simulink library "generator_lib"  (Simulink 7.8)
settings: Solver=ode45  StartTime=0.0  StopTime=10.0  RelTol=1e-3
undefined symbols (not defined in the file): dfilt, DiscIntNeverNeededParam, fdesignblkfcn, gcbh, ph, Ts
libraries: simulink x91, rtio_opalrt_common x84, powerlib x51, simulink_extras x21, discretizing x14, rteventslib x14, dsparch4 x14, powerlib_extras x4
(part 2 of 10)

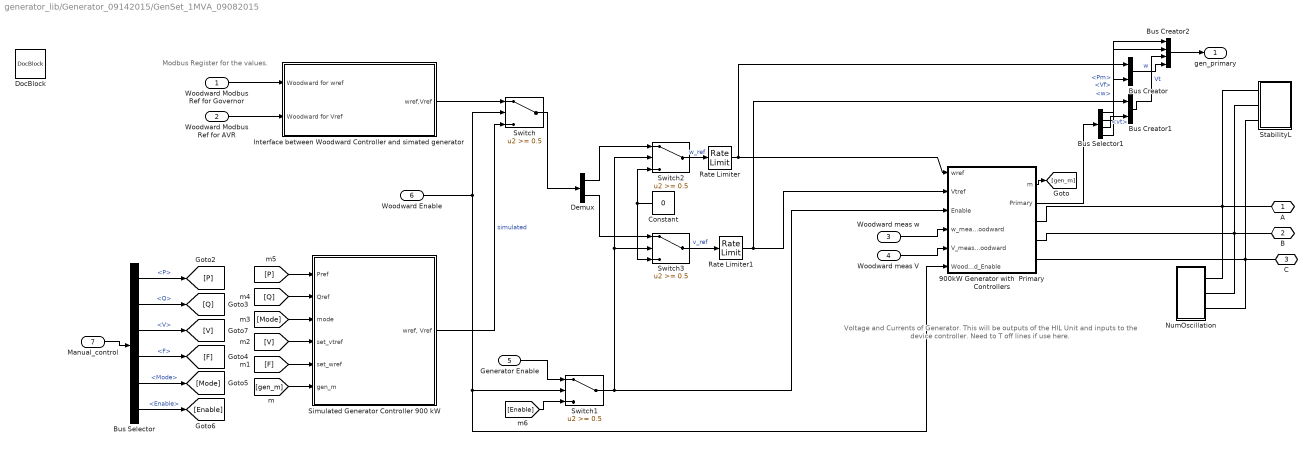
== system generator_lib/Generator_09142015/GenSet_1MVA_09082015 ==
  note: Voltage and Currents of Generator.
      | This will be outputs of the HIL Unit
      | and inputs to the device controller.
      | Need to T off lines if use here.
  note: Modbus Register for the values.
  Woodward Modbus Ref for Governor : Inport
  Woodward Modbus Ref for AVR : Inport  Port=2
  Woodward meas w : Inport  Port=3
  Woodward meas V : Inport  Port=4
  Generator Enable : Inport  Port=5
  Woodward Enable : Inport  Port=6
  Manual_control : Inport  Port=7
  900kW Generator with  Primary Controllers : Subsystem
  Bus Creator : BusCreator  Inputs=2
  Bus Creator1 : BusCreator  Inputs=2
  Bus Creator2 : BusCreator
  Bus Selector : BusSelector  OutputSignals=P,Q,V,F,Mode,Enable
  Bus Selector1 : BusSelector  OutputSignals=Pm,Vf,vt,w
  Constant : Constant  Value=0
  Demux : Demux  Outputs=2
  DocBlock : simulink/Model-Wide Utilities/DocBlock  DocumentType=Text
  Interface between Woodward Controller and simated generator : Subsystem
  NumOscillation : Subsystem
  Rate Limiter : RateLimiter  RisingSlewLimit=0.5  FallingSlewLimit=-0.5  SampleTimeMode=inherited
  Rate Limiter1 : RateLimiter  RisingSlewLimit=0.5  FallingSlewLimit=-0.5  SampleTimeMode=inherited
  Simulated Generator Controller 900 kW : Subsystem
  StabilityL : Subsystem  mask{v=460, kVA=50, pf=1}
  Switch{,1..3} (4 alike) : Switch  Threshold=0.5
  A : PMIOPort  Port=1  Side=Right
  B : PMIOPort  Port=2  Side=Right
  C : PMIOPort  Port=3  Side=Right
  gen_primary : Outport
  wires:
  Woodward Enable/1 -> 900kW Generator with  Primary Controllers/6(Woodward_Enable), Switch1/2, Switch/2
  Rate Limiter1/1 -> Bus Creator1/1, 900kW Generator with  Primary Controllers/2(Vtref)
  Rate Limiter/1 -> Bus Creator/1, 900kW Generator with  Primary Controllers/1(wref)
  Bus Creator2/1 -> gen_primary/1
  Bus Creator/1 -> Bus Creator2/4  "w"
  Bus Creator1/1 -> Bus Creator2/3  "Vt"
  Bus Selector1/1 -> Bus Creator2/1  "<Pm>"
  Bus Selector1/2 -> Bus Creator2/2  "<Vf>"
  Bus Selector1/4 -> Bus Creator/2  "<w>"
  Bus Selector1/3 -> Bus Creator1/2  "<vt>"
  Switch3/1 -> Rate Limiter1/1  "v_ref"
  Constant/1 -> Switch2/3, Switch3/3
  Demux/2 -> Switch3/1
  Demux/1 -> Switch2/1
  Switch2/1 -> Rate Limiter/1  "w_ref"
  Switch1/1 -> Switch3/2, Switch2/2, 900kW Generator with  Primary Controllers/3(Enable)
  [Enable] -> Switch1/3
  Generator Enable/1 -> Switch1/1
  900kW Generator with  Primary Controllers/2(Primary) -> Bus Selector1/1
  Bus Selector/6 -> [Enable]  "<Enable>"
  Woodward meas V/1 -> 900kW Generator with  Primary Controllers/5(V_meas_Woodward)
  Woodward meas w/1 -> 900kW Generator with  Primary Controllers/4(w_meas_Woodward)
  Woodward Modbus Ref for AVR/1 -> Interface between Woodward Controller and simated generator/2(Woodward for Vref)
  Woodward Modbus Ref for Governor/1 -> Interface between Woodward Controller and simated generator/1(Woodward for wref)
  Switch/1 -> Demux/1
  Interface between Woodward Controller and simated generator/1(wref,Vref) -> Switch/1
  900kW Generator with  Primary Controllers/1(m) -> [gen_m]
  Simulated Generator Controller 900 kW/1("wref, Vref") -> Switch/3  "simulated"
  Manual_control/1 -> Bus Selector/1
  Bus Selector/1 -> [P]  "<P>"
  Bus Selector/2 -> [Q]  "<Q>"
  Bus Selector/3 -> [V]  "<V>"
  Bus Selector/4 -> [F]  "<F>"
  Bus Selector/5 -> [Mode]  "<Mode>"
  [gen_m] -> Simulated Generator Controller 900 kW/6(gen_m)
  [P] -> Simulated Generator Controller 900 kW/1(Pref)
  [Q] -> Simulated Generator Controller 900 kW/2(Qref)
  [Mode] -> Simulated Generator Controller 900 kW/3(mode)
  [V] -> Simulated Generator Controller 900 kW/4(set_vtref)
  [F] -> Simulated Generator Controller 900 kW/5(set_wref)
  connections:
  NumOscillation/LConn3 -- 900kW Generator with  Primary Controllers/RConn3 -- C/RConn1 -- StabilityL/LConn3
  NumOscillation/LConn2 -- B/RConn1 -- 900kW Generator with  Primary Controllers/RConn2 -- StabilityL/LConn2
  NumOscillation/LConn1 -- 900kW Generator with  Primary Controllers/RConn1 -- A/RConn1 -- StabilityL/LConn1

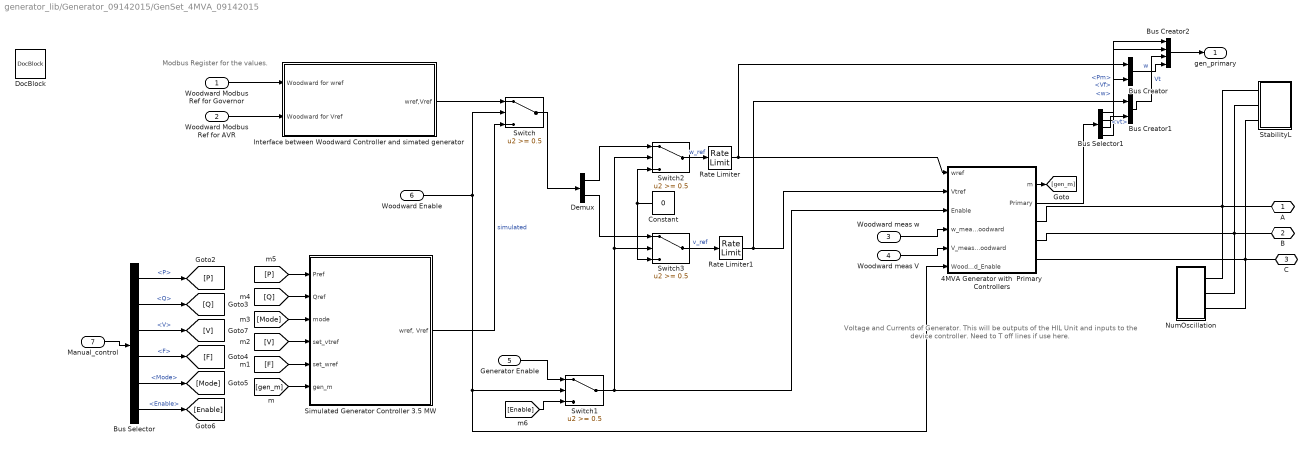
== system generator_lib/Generator_09142015/GenSet_4MVA_09142015 ==
  note: Voltage and Currents of Generator.
      | This will be outputs of the HIL Unit
      | and inputs to the device controller.
      | Need to T off lines if use here.
  note: Modbus Register for the values.
  Woodward Modbus Ref for Governor : Inport
  Woodward Modbus Ref for AVR : Inport  Port=2
  Woodward meas w : Inport  Port=3
  Woodward meas V : Inport  Port=4
  Generator Enable : Inport  Port=5
  Woodward Enable : Inport  Port=6
  Manual_control : Inport  Port=7
  4MVA Generator with  Primary Controllers : Subsystem
  Bus Creator : BusCreator  Inputs=2
  Bus Creator1 : BusCreator  Inputs=2
  Bus Creator2 : BusCreator
  Bus Selector : BusSelector  OutputSignals=P,Q,V,F,Mode,Enable
  Bus Selector1 : BusSelector  OutputSignals=Pm,Vf,vt,w
  Constant : Constant  Value=0
  Demux : Demux  Outputs=2
  DocBlock : simulink/Model-Wide Utilities/DocBlock  DocumentType=Text
  Interface between Woodward Controller and simated generator : Subsystem
  NumOscillation : Subsystem
  Rate Limiter : RateLimiter  RisingSlewLimit=0.5  FallingSlewLimit=-0.5  SampleTimeMode=inherited
  Rate Limiter1 : RateLimiter  RisingSlewLimit=0.5  FallingSlewLimit=-0.5  SampleTimeMode=inherited
  Simulated Generator Controller 3.5 MW : Subsystem
  StabilityL : Subsystem  mask{v=13800, kVA=300, pf=1}
  Switch{,1..3} (4 alike) : Switch  Threshold=0.5
  A : PMIOPort  Port=1  Side=Right
  B : PMIOPort  Port=2  Side=Right
  C : PMIOPort  Port=3  Side=Right
  gen_primary : Outport
  wires:
  Woodward Enable/1 -> 4MVA Generator with  Primary Controllers/6(Woodward_Enable), Switch1/2, Switch/2
  Rate Limiter1/1 -> Bus Creator1/1, 4MVA Generator with  Primary Controllers/2(Vtref)
  Rate Limiter/1 -> Bus Creator/1, 4MVA Generator with  Primary Controllers/1(wref)
  Bus Creator2/1 -> gen_primary/1
  Bus Creator/1 -> Bus Creator2/4  "w"
  Bus Creator1/1 -> Bus Creator2/3  "Vt"
  Bus Selector1/1 -> Bus Creator2/1  "<Pm>"
  Bus Selector1/2 -> Bus Creator2/2  "<Vf>"
  Bus Selector1/4 -> Bus Creator/2  "<w>"
  Bus Selector1/3 -> Bus Creator1/2  "<vt>"
  Switch3/1 -> Rate Limiter1/1  "v_ref"
  Constant/1 -> Switch2/3, Switch3/3
  Demux/2 -> Switch3/1
  Demux/1 -> Switch2/1
  Switch2/1 -> Rate Limiter/1  "w_ref"
  Switch1/1 -> Switch3/2, Switch2/2, 4MVA Generator with  Primary Controllers/3(Enable)
  [Enable] -> Switch1/3
  Generator Enable/1 -> Switch1/1
  4MVA Generator with  Primary Controllers/2(Primary) -> Bus Selector1/1
  Bus Selector/6 -> [Enable]  "<Enable>"
  Woodward meas V/1 -> 4MVA Generator with  Primary Controllers/5(V_meas_Woodward)
  Woodward meas w/1 -> 4MVA Generator with  Primary Controllers/4(w_meas_Woodward)
  Woodward Modbus Ref for AVR/1 -> Interface between Woodward Controller and simated generator/2(Woodward for Vref)
  Woodward Modbus Ref for Governor/1 -> Interface between Woodward Controller and simated generator/1(Woodward for wref)
  Switch/1 -> Demux/1
  Interface between Woodward Controller and simated generator/1(wref,Vref) -> Switch/1
  4MVA Generator with  Primary Controllers/1(m) -> [gen_m]
  Simulated Generator Controller 3.5 MW/1("wref, Vref") -> Switch/3  "simulated"
  Manual_control/1 -> Bus Selector/1
  Bus Selector/1 -> [P]  "<P>"
  Bus Selector/2 -> [Q]  "<Q>"
  Bus Selector/3 -> [V]  "<V>"
  Bus Selector/4 -> [F]  "<F>"
  Bus Selector/5 -> [Mode]  "<Mode>"
  [gen_m] -> Simulated Generator Controller 3.5 MW/6(gen_m)
  [P] -> Simulated Generator Controller 3.5 MW/1(Pref)
  [Q] -> Simulated Generator Controller 3.5 MW/2(Qref)
  [Mode] -> Simulated Generator Controller 3.5 MW/3(mode)
  [V] -> Simulated Generator Controller 3.5 MW/4(set_vtref)
  [F] -> Simulated Generator Controller 3.5 MW/5(set_wref)
  connections:
  NumOscillation/LConn3 -- 4MVA Generator with  Primary Controllers/RConn3 -- C/RConn1 -- StabilityL/LConn3
  NumOscillation/LConn2 -- B/RConn1 -- 4MVA Generator with  Primary Controllers/RConn2 -- StabilityL/LConn2
  NumOscillation/LConn1 -- 4MVA Generator with  Primary Controllers/RConn1 -- A/RConn1 -- StabilityL/LConn1

== system generator_lib/Generator_09142015/Woodward Inputs ==
  note: There will need to be a
      | new scaling factor to use
      | the current cards (0-1A)
  note: GR1 A AOUT (CH00-15)
  note: For 120 => 12Vout / 170Vpk
      | For 480 => 12Vout / 391Vpk
      | For 13.8kv => 12Vout / 11268Vpk
  note: 6Vout / ( 900,000W / 391 Vpk)
  MPU1_speed : Inport
  Generator1_Voltage : Inport  Port=2
  Generator1_Current : Inport  Port=3
  Mains1_Voltage : Inport  Port=4
  Mains1_Current : Inport  Port=5
  MPU2_speed : Inport  Port=6
  Generator2_Voltage : Inport  Port=7
  Generator2_Current : Inport  Port=8
  Mains2_Voltage : Inport  Port=9
  Mains2_Current : Inport  Port=10
  AnalogOut : rtio_opalrt_common/AnalogOut  CtrlName='OpCtrl'  portNb=1  FcnNos=Slot 1 Module A Subsection 1  size=16  maxcount=8  count=8  numchan=8  israngeinput=off  voltagerange=[-16 ... 16]  slot=0  side=0  mismatch=0  slotside=Slot_1_Module_A
      settings: AttributesFormatString=%<CtrlName>
  AnalogOut1 : rtio_opalrt_common/AnalogOut  CtrlName='OpCtrl'  portNb=2  FcnNos=Slot 1 Module A Subsection 2  size=16  maxcount=8  count=8  numchan=8  israngeinput=off  voltagerange=[-16 ... 16]  slot=0  side=0  mismatch=0  slotside=Slot_1_Module_A
      settings: AttributesFormatString=%<CtrlName>
  AnalogOut2 : rtio_opalrt_common/AnalogOut  CtrlName='OpCtrl'  portNb=3  FcnNos=Slot 2 Module A Subsection 1  size=16  maxcount=8  count=8  numchan=8  israngeinput=off  voltagerange=[-16 ... 16]  slot=1  side=0  mismatch=0  slotside=Slot_2_Module_A
      settings: AttributesFormatString=%<CtrlName>
  AnalogOut3 : rtio_opalrt_common/AnalogOut  CtrlName='OpCtrl'  portNb=4  FcnNos=Slot 2 Module A Subsection 2  size=16  maxcount=8  count=8  numchan=8  israngeinput=off  voltagerange=[-16 ... 16]  slot=1  side=0  mismatch=0  slotside=Slot_2_Module_A
      settings: AttributesFormatString=%<CtrlName>
  Demux : Demux  Outputs=2
  Demux{1..5,7..9} (8 alike) : Demux  Outputs=3
  Demux6 : Demux  Outputs=2
  Gain : Gain  Gain=15/391
  Gain1 : Gain  Gain=15/11268
  Gain2 : Gain  Gain=15/(900000/391)
  Gain3 : Gain  Gain=15/(900000/11268)
  Gain4 : Gain  Gain=15/11268
  Gain5 : Gain  Gain=15/11268
  Gain6 : Gain  Gain=15/(900000/391)
  Gain7 : Gain  Gain=15/(900000/11268)
  Mux{,1,3..4} (4 alike) : Mux  Inputs=8
  Mux2 : Mux  Inputs=2
  Mux5 : Mux  Inputs=2
  Speed_System : Subsystem
  Speed_System1 : Subsystem
  Terminator{,1..3} (4 alike) : Terminator
  wires:
  Demux9/3 -> Mux3/8
  Demux9/2 -> Mux3/7
  Demux9/1 -> Mux3/6
  Gain6/1 -> Demux9/1
  Demux8/1 -> Mux3/5
  Gain7/1 -> Demux8/1
  Mains2_Current/1 -> Gain7/1
  Generator2_Current/1 -> Gain6/1
  Speed_System1/1(Out1) -> Mux1/6
  MPU2_speed/1 -> Speed_System1/1(In1)
  Generator2_Voltage/1 -> Gain4/1
  Mains2_Voltage/1 -> Gain5/1
  Gain4/1 -> Demux4/1
  Gain5/1 -> Demux5/1
  Demux7/1 -> Mux3/1
  Gain3/1 -> Demux7/1
  Mains1_Current/1 -> Gain3/1
  Demux3/3 -> Mux3/4
  Demux3/2 -> Mux3/3
  Demux3/1 -> Mux3/2
  Gain2/1 -> Demux3/1
  AnalogOut2/1 -> Terminator2/1
  AnalogOut3/1 -> Terminator3/1
  Demux6/1 -> AnalogOut2/1
  Demux6/2 -> AnalogOut3/1
  Mux3/1 -> Mux5/1
  Mux4/1 -> Mux5/2
  Mux5/1 -> Demux6/1
  Demux5/3 -> Mux1/4
  Demux5/2 -> Mux1/3
  Demux5/1 -> Mux1/2
  Demux4/3 -> Mux1/1
  Demux4/2 -> Mux/8
  Demux4/1 -> Mux/7
  Speed_System/1(Out1) -> Mux1/5
  Demux2/3 -> Mux/6
  Demux2/2 -> Mux/5
  Demux2/1 -> Mux/4
  Demux1/3 -> Mux/3
  Demux1/2 -> Mux/2
  Demux1/1 -> Mux/1
  AnalogOut/1 -> Terminator/1
  AnalogOut1/1 -> Terminator1/1
  Demux/1 -> AnalogOut/1
  Demux/2 -> AnalogOut1/1
  Generator1_Voltage/1 -> Gain/1
  Mux/1 -> Mux2/1
  Mux1/1 -> Mux2/2
  Mux2/1 -> Demux/1
  Mains1_Voltage/1 -> Gain1/1
  Gain/1 -> Demux1/1
  Gain1/1 -> Demux2/1
  Generator1_Current/1 -> Gain2/1
  MPU1_speed/1 -> Speed_System/1(In1)

== system generator_lib/Generator_09142015/Woodward Outputs ==
  Digital Output : Inport
  DIO Enable : Inport  Port=2
  Bias Enable : Inport  Port=3
  Bus Creator1 : BusCreator  Inputs=3
  DIO - Gr3 : Subsystem
  DIO - Woodward : Subsystem
  DOUT type config : Subsystem
  OpCtrl : rtio_opalrt_common/OpCtrl  CtrlName='OpCtrl'  boardid=0  BitstreamFilename=VC707_2-EX-0001-2_2_6_61-32AIO16DIO16DIOSel-01-01.bin  numconfig=-1  mode=Master  externalClock=off  decimRtsi=0  calibIO=off  SampleTime=0  loadinport=-1  BoardType=VC707  SecondaryPresent=off  sync_type=Audio
  PWM IO - Gr3 : Subsystem
  TSDIO - Gr3 : Subsystem
  Woodward Primary Inputs : Subsystem
  Error : Outport
  IDs : Outport  Port=2
  Digital Inputs : Outport  Port=3
  Gen1 Gov and AVR : Outport  Port=4
  Gen2 Gov and AVR : Outport  Port=5
  Gen1 Fuel Enable : Outport  Port=6
  Gen1 GCB : Outport  Port=7
  Gen1 MCB : Outport  Port=8
  Gen2 Fuel Enable : Outport  Port=9
  Gen2 GCB : Outport  Port=10
  Gen2 MCB : Outport  Port=11
  wires:
  DIO - Woodward/7(Gen2 MCB) -> Gen2 MCB/1
  DIO - Woodward/5(Gen2 Fuel Enable) -> Gen2 Fuel Enable/1
  DIO - Woodward/6(Gen2 GCB) -> Gen2 GCB/1
  DIO - Woodward/1(Gen1 Fuel Enable) -> Gen1 Fuel Enable/1
  DIO - Woodward/3(Gen1 MCB) -> Gen1 MCB/1
  DIO - Woodward/2(Gen1 GCB) -> Gen1 GCB/1
  Digital Output/1 -> TSDIO - Gr3/1(TSDout), PWM IO - Gr3/1(PWMOut), DIO - Woodward/2(Din_sim)
  Bias Enable/1 -> Woodward Primary Inputs/1(Bias-ctrl)
  Woodward Primary Inputs/2(Gen2 Gov and AVR) -> Gen2 Gov and AVR/1
  Woodward Primary Inputs/1(Gen1 Gov and AVR) -> Gen1 Gov and AVR/1
  DIO Enable/1 -> DIO - Woodward/4(control1), DIO - Woodward/3(control)
  Bus Creator1/1 -> Digital Inputs/1
  DIO - Gr3/1(DIn) -> DIO - Woodward/1(Din_Wood1), Bus Creator1/1  "DIN"
  TSDIO - Gr3/1(TSDin) -> Bus Creator1/2  "TSDIN"
  PWM IO - Gr3/1(PWMIn) -> Bus Creator1/3  "PWMIN"
  DIO - Woodward/4(DIn1) -> DIO - Gr3/1(Dout)
  OpCtrl/2 -> IDs/1
  OpCtrl/1 -> Error/1

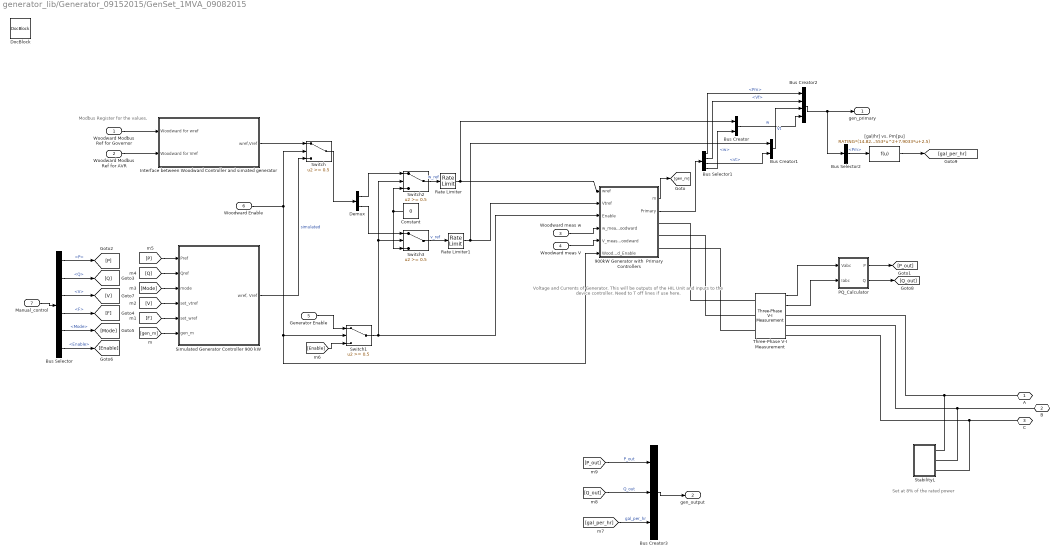
== system generator_lib/Generator_09152015/GenSet_1MVA_09082015 ==
  note: Set at 8% of the rated power
  note: Voltage and Currents of Generator.
      | This will be outputs of the HIL Unit
      | and inputs to the device controller.
      | Need to T off lines if use here.
  note: Modbus Register for the values.
  Woodward Modbus Ref for Governor : Inport
  Woodward Modbus Ref for AVR : Inport  Port=2
  Woodward meas w : Inport  Port=3
  Woodward meas V : Inport  Port=4
  Generator Enable : Inport  Port=5
  Woodward Enable : Inport  Port=6
  Manual_control : Inport  Port=7
  900kW Generator with  Primary Controllers : Subsystem
  Bus Creator : BusCreator  Inputs=2
  Bus Creator1 : BusCreator  Inputs=2
  Bus Creator2 : BusCreator
  Bus Creator3 : BusCreator  Inputs=3
  Bus Selector : BusSelector  OutputSignals=P,Q,V,F,Mode,Enable
  Bus Selector1 : BusSelector  OutputSignals=Pm,Vf,vt,w
  Bus Selector2 : BusSelector  OutputSignals=Pm
  Constant : Constant  Value=0
  Demux : Demux  Outputs=2
  DocBlock : simulink/Model-Wide Utilities/DocBlock  DocumentType=Text
  Interface between Woodward Controller and simated generator : Subsystem
  PQ_Calculator : Subsystem
  Rate Limiter : RateLimiter  RisingSlewLimit=0.5  FallingSlewLimit=-0.5  SampleTimeMode=inherited
  Rate Limiter1 : RateLimiter  RisingSlewLimit=0.5  FallingSlewLimit=-0.5  SampleTimeMode=inherited
  Simulated Generator Controller 900 kW : Subsystem
  StabilityL : Subsystem  mask{v=460, kVA=80, pf=1}
  Switch{,1..3} (4 alike) : Switch  Threshold=0.5
  Three-Phase V-I Measurement : powerlib/Measurements/Three-Phase V-I Measurement  VoltageMeasurement=phase-to-ground  SetLabelV=off  LabelV=Vabc  Vpu=off  VpuLL=off  CurrentMeasurement=yes  SetLabelI=off  LabelI=Iabc  Ipu=off  Pbase=100e6  Vbase=500e3  OutputType=Complex  PhasorSimulation=off  PSBequivalent=0
  "[gal/hr] vs. Pm[pu]" : Fcn  Expr=RATING*(14.827*u^4-27.253*u^3+15.553*u^2+7.9033*u+2.5)  mask{RATING=1}
      mask prompts: RATING "Rating [MW]"
      mask help: This block computes the gal/hr vs Pm[pu] of a generator of a given rating [MW].
  A : PMIOPort  Port=1  Side=Right
  B : PMIOPort  Port=2  Side=Right
  C : PMIOPort  Port=3  Side=Right
  gen_primary : Outport
  gen_output : Outport  Port=2
  wires:
  Bus Creator3/1 -> gen_output/1
  [gal_per_hr] -> Bus Creator3/3  "gal_per_hr"
  [Q_out] -> Bus Creator3/2  "Q_out"
  [P_out] -> Bus Creator3/1  "P_out"
  Bus Selector2/1 -> "[gal/hr] vs. Pm[pu]"/1  "<Pm>"
  "[gal/hr] vs. Pm[pu]"/1 -> [gal_per_hr]
  Three-Phase V-I Measurement/2 -> PQ_Calculator/2(Iabc)
  Three-Phase V-I Measurement/1 -> PQ_Calculator/1(Vabc)
  PQ_Calculator/2(Q) -> [Q_out]
  PQ_Calculator/1(P) -> [P_out]
  Woodward Enable/1 -> 900kW Generator with  Primary Controllers/6(Woodward_Enable), Switch1/2, Switch/2
  Rate Limiter1/1 -> Bus Creator1/1, 900kW Generator with  Primary Controllers/2(Vtref)
  Rate Limiter/1 -> Bus Creator/1, 900kW Generator with  Primary Controllers/1(wref)
  Bus Creator2/1 -> Bus Selector2/1, gen_primary/1
  Bus Creator/1 -> Bus Creator2/4  "w"
  Bus Creator1/1 -> Bus Creator2/3  "Vt"
  Bus Selector1/1 -> Bus Creator2/1  "<Pm>"
  Bus Selector1/2 -> Bus Creator2/2  "<Vf>"
  Bus Selector1/4 -> Bus Creator/2  "<w>"
  Bus Selector1/3 -> Bus Creator1/2  "<vt>"
  Switch3/1 -> Rate Limiter1/1  "v_ref"
  Constant/1 -> Switch2/3, Switch3/3
  Demux/2 -> Switch3/1
  Demux/1 -> Switch2/1
  Switch2/1 -> Rate Limiter/1  "w_ref"
  Switch1/1 -> Switch3/2, Switch2/2, 900kW Generator with  Primary Controllers/3(Enable)
  [Enable] -> Switch1/3
  Generator Enable/1 -> Switch1/1
  900kW Generator with  Primary Controllers/2(Primary) -> Bus Selector1/1
  Bus Selector/6 -> [Enable]  "<Enable>"
  Woodward meas V/1 -> 900kW Generator with  Primary Controllers/5(V_meas_Woodward)
  Woodward meas w/1 -> 900kW Generator with  Primary Controllers/4(w_meas_Woodward)
  Woodward Modbus Ref for AVR/1 -> Interface between Woodward Controller and simated generator/2(Woodward for Vref)
  Woodward Modbus Ref for Governor/1 -> Interface between Woodward Controller and simated generator/1(Woodward for wref)
  Switch/1 -> Demux/1
  Interface between Woodward Controller and simated generator/1(wref,Vref) -> Switch/1
  900kW Generator with  Primary Controllers/1(m) -> [gen_m]
  Simulated Generator Controller 900 kW/1("wref, Vref") -> Switch/3  "simulated"
  Manual_control/1 -> Bus Selector/1
  Bus Selector/1 -> [P]  "<P>"
  Bus Selector/2 -> [Q]  "<Q>"
  Bus Selector/3 -> [V]  "<V>"
  Bus Selector/4 -> [F]  "<F>"
  Bus Selector/5 -> [Mode]  "<Mode>"
  [gen_m] -> Simulated Generator Controller 900 kW/6(gen_m)
  [P] -> Simulated Generator Controller 900 kW/1(Pref)
  [Q] -> Simulated Generator Controller 900 kW/2(Qref)
  [Mode] -> Simulated Generator Controller 900 kW/3(mode)
  [V] -> Simulated Generator Controller 900 kW/4(set_vtref)
  [F] -> Simulated Generator Controller 900 kW/5(set_wref)
  connections:
  StabilityL/LConn3 -- Three-Phase V-I Measurement/RConn3 -- C/RConn1
  StabilityL/LConn2 -- Three-Phase V-I Measurement/RConn2 -- B/RConn1
  StabilityL/LConn1 -- Three-Phase V-I Measurement/RConn1 -- A/RConn1
  Three-Phase V-I Measurement/LConn1 -- 900kW Generator with  Primary Controllers/RConn1
  Three-Phase V-I Measurement/LConn2 -- 900kW Generator with  Primary Controllers/RConn2
  Three-Phase V-I Measurement/LConn3 -- 900kW Generator with  Primary Controllers/RConn3

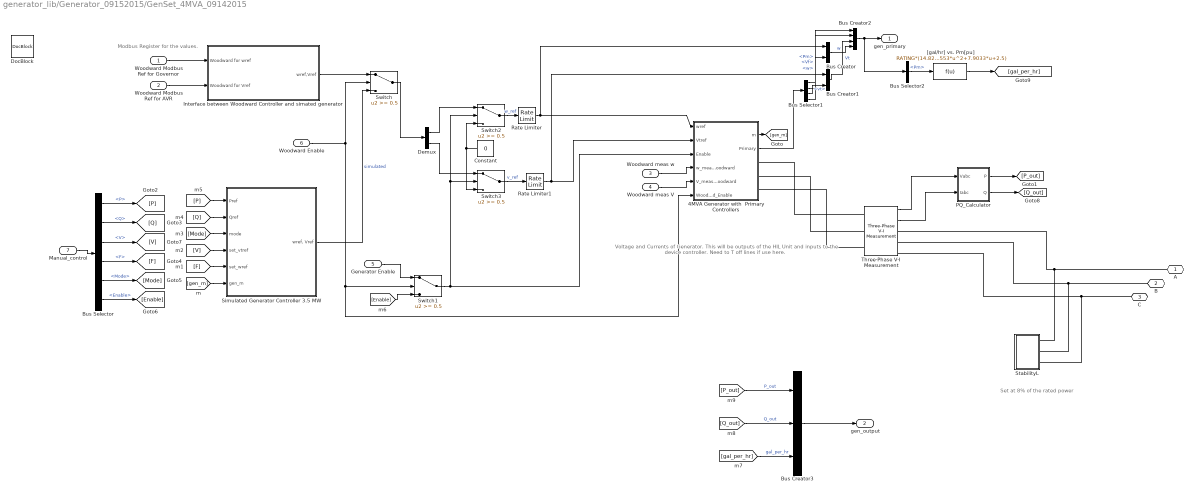
== system generator_lib/Generator_09152015/GenSet_4MVA_09142015 ==
  note: Set at 8% of the rated power
  note: Voltage and Currents of Generator.
      | This will be outputs of the HIL Unit
      | and inputs to the device controller.
      | Need to T off lines if use here.
  note: Modbus Register for the values.
  Woodward Modbus Ref for Governor : Inport
  Woodward Modbus Ref for AVR : Inport  Port=2
  Woodward meas w : Inport  Port=3
  Woodward meas V : Inport  Port=4
  Generator Enable : Inport  Port=5
  Woodward Enable : Inport  Port=6
  Manual_control : Inport  Port=7
  4MVA Generator with  Primary Controllers : Subsystem
  Bus Creator : BusCreator  Inputs=2
  Bus Creator1 : BusCreator  Inputs=2
  Bus Creator2 : BusCreator
  Bus Creator3 : BusCreator  Inputs=3
  Bus Selector : BusSelector  OutputSignals=P,Q,V,F,Mode,Enable
  Bus Selector1 : BusSelector  OutputSignals=Pm,Vf,vt,w
  Bus Selector2 : BusSelector  OutputSignals=Pm
  Constant : Constant  Value=0
  Demux : Demux  Outputs=2
  DocBlock : simulink/Model-Wide Utilities/DocBlock  DocumentType=Text
  Interface between Woodward Controller and simated generator : Subsystem
  PQ_Calculator : Subsystem
  Rate Limiter : RateLimiter  RisingSlewLimit=0.5  FallingSlewLimit=-0.5  SampleTimeMode=inherited
  Rate Limiter1 : RateLimiter  RisingSlewLimit=0.5  FallingSlewLimit=-0.5  SampleTimeMode=inherited
  Simulated Generator Controller 3.5 MW : Subsystem
  StabilityL : Subsystem  mask{v=13800, kVA=320, pf=1}
  Switch{,1..3} (4 alike) : Switch  Threshold=0.5
  Three-Phase V-I Measurement : powerlib/Measurements/Three-Phase V-I Measurement  VoltageMeasurement=phase-to-ground  SetLabelV=off  LabelV=Vabc  Vpu=off  VpuLL=off  CurrentMeasurement=yes  SetLabelI=off  LabelI=Iabc  Ipu=off  Pbase=100e6  Vbase=500e3  OutputType=Complex  PhasorSimulation=off  PSBequivalent=0
  "[gal/hr] vs. Pm[pu]" : Fcn  Expr=RATING*(14.827*u^4-27.253*u^3+15.553*u^2+7.9033*u+2.5)  mask{RATING=4}
      mask prompts: RATING "Rating [MW]"
      mask help: This block computes the gal/hr vs Pm[pu] of a generator of a given rating [MW].
  A : PMIOPort  Port=1  Side=Right
  B : PMIOPort  Port=2  Side=Right
  C : PMIOPort  Port=3  Side=Right
  gen_primary : Outport
  gen_output : Outport  Port=2
  wires:
  Bus Creator3/1 -> gen_output/1
  [gal_per_hr] -> Bus Creator3/3  "gal_per_hr"
  [Q_out] -> Bus Creator3/2  "Q_out"
  [P_out] -> Bus Creator3/1  "P_out"
  Bus Selector2/1 -> "[gal/hr] vs. Pm[pu]"/1  "<Pm>"
  "[gal/hr] vs. Pm[pu]"/1 -> [gal_per_hr]
  Three-Phase V-I Measurement/2 -> PQ_Calculator/2(Iabc)
  Three-Phase V-I Measurement/1 -> PQ_Calculator/1(Vabc)
  PQ_Calculator/2(Q) -> [Q_out]
  PQ_Calculator/1(P) -> [P_out]
  Woodward Enable/1 -> 4MVA Generator with  Primary Controllers/6(Woodward_Enable), Switch1/2, Switch/2
  Rate Limiter1/1 -> Bus Creator1/1, 4MVA Generator with  Primary Controllers/2(Vtref)
  Rate Limiter/1 -> Bus Creator/1, 4MVA Generator with  Primary Controllers/1(wref)
  Bus Creator2/1 -> Bus Selector2/1, gen_primary/1
  Bus Creator/1 -> Bus Creator2/4  "w"
  Bus Creator1/1 -> Bus Creator2/3  "Vt"
  Bus Selector1/1 -> Bus Creator2/1  "<Pm>"
  Bus Selector1/2 -> Bus Creator2/2  "<Vf>"
  Bus Selector1/4 -> Bus Creator/2  "<w>"
  Bus Selector1/3 -> Bus Creator1/2  "<vt>"
  Switch3/1 -> Rate Limiter1/1  "v_ref"
  Constant/1 -> Switch2/3, Switch3/3
  Demux/2 -> Switch3/1
  Demux/1 -> Switch2/1
  Switch2/1 -> Rate Limiter/1  "w_ref"
  Switch1/1 -> Switch3/2, Switch2/2, 4MVA Generator with  Primary Controllers/3(Enable)
  [Enable] -> Switch1/3
  Generator Enable/1 -> Switch1/1
  4MVA Generator with  Primary Controllers/2(Primary) -> Bus Selector1/1
  Bus Selector/6 -> [Enable]  "<Enable>"
  Woodward meas V/1 -> 4MVA Generator with  Primary Controllers/5(V_meas_Woodward)
  Woodward meas w/1 -> 4MVA Generator with  Primary Controllers/4(w_meas_Woodward)
  Woodward Modbus Ref for AVR/1 -> Interface between Woodward Controller and simated generator/2(Woodward for Vref)
  Woodward Modbus Ref for Governor/1 -> Interface between Woodward Controller and simated generator/1(Woodward for wref)
  Switch/1 -> Demux/1
  Interface between Woodward Controller and simated generator/1(wref,Vref) -> Switch/1
  4MVA Generator with  Primary Controllers/1(m) -> [gen_m]
  Simulated Generator Controller 3.5 MW/1("wref, Vref") -> Switch/3  "simulated"
  Manual_control/1 -> Bus Selector/1
  Bus Selector/1 -> [P]  "<P>"
  Bus Selector/2 -> [Q]  "<Q>"
  Bus Selector/3 -> [V]  "<V>"
  Bus Selector/4 -> [F]  "<F>"
  Bus Selector/5 -> [Mode]  "<Mode>"
  [gen_m] -> Simulated Generator Controller 3.5 MW/6(gen_m)
  [P] -> Simulated Generator Controller 3.5 MW/1(Pref)
  [Q] -> Simulated Generator Controller 3.5 MW/2(Qref)
  [Mode] -> Simulated Generator Controller 3.5 MW/3(mode)
  [V] -> Simulated Generator Controller 3.5 MW/4(set_vtref)
  [F] -> Simulated Generator Controller 3.5 MW/5(set_wref)
  connections:
  StabilityL/LConn3 -- Three-Phase V-I Measurement/RConn3 -- C/RConn1
  StabilityL/LConn2 -- Three-Phase V-I Measurement/RConn2 -- B/RConn1
  StabilityL/LConn1 -- Three-Phase V-I Measurement/RConn1 -- A/RConn1
  Three-Phase V-I Measurement/LConn1 -- 4MVA Generator with  Primary Controllers/RConn1
  Three-Phase V-I Measurement/LConn2 -- 4MVA Generator with  Primary Controllers/RConn2
  Three-Phase V-I Measurement/LConn3 -- 4MVA Generator with  Primary Controllers/RConn3

== system generator_lib/Generator_09152015/Woodward Inputs ==
  note: There will need to be a
      | new scaling factor to use
      | the current cards (0-1A)
  note: GR1 A AOUT (CH00-15)
  note: For 120 => 12Vout / 170Vpk
      | For 480 => 12Vout / 391Vpk
      | For 13.8kv => 12Vout / 11268Vpk
  note: 6Vout / ( 900,000W / 391 Vpk)
  MPU1_speed : Inport
  Generator1_Voltage : Inport  Port=2
  Generator1_Current : Inport  Port=3
  Mains1_Voltage : Inport  Port=4
  Mains1_Current : Inport  Port=5
  MPU2_speed : Inport  Port=6
  Generator2_Voltage : Inport  Port=7
  Generator2_Current : Inport  Port=8
  Mains2_Voltage : Inport  Port=9
  Mains2_Current : Inport  Port=10
  AnalogOut : rtio_opalrt_common/AnalogOut  CtrlName='OpCtrl'  portNb=1  FcnNos=Slot 1 Module A Subsection 1  size=16  maxcount=8  count=8  numchan=8  israngeinput=off  voltagerange=[-16 ... 16]  slot=0  side=0  mismatch=0  slotside=Slot_1_Module_A
      settings: AttributesFormatString=%<CtrlName>
  AnalogOut1 : rtio_opalrt_common/AnalogOut  CtrlName='OpCtrl'  portNb=2  FcnNos=Slot 1 Module A Subsection 2  size=16  maxcount=8  count=8  numchan=8  israngeinput=off  voltagerange=[-16 ... 16]  slot=0  side=0  mismatch=0  slotside=Slot_1_Module_A
      settings: AttributesFormatString=%<CtrlName>
  AnalogOut2 : rtio_opalrt_common/AnalogOut  CtrlName='OpCtrl'  portNb=3  FcnNos=Slot 2 Module A Subsection 1  size=16  maxcount=8  count=8  numchan=8  israngeinput=off  voltagerange=[-16 ... 16]  slot=1  side=0  mismatch=0  slotside=Slot_2_Module_A
      settings: AttributesFormatString=%<CtrlName>
  AnalogOut3 : rtio_opalrt_common/AnalogOut  CtrlName='OpCtrl'  portNb=4  FcnNos=Slot 2 Module A Subsection 2  size=16  maxcount=8  count=8  numchan=8  israngeinput=off  voltagerange=[-16 ... 16]  slot=1  side=0  mismatch=0  slotside=Slot_2_Module_A
      settings: AttributesFormatString=%<CtrlName>
  Demux : Demux  Outputs=2
  Demux{1..5,7..9} (8 alike) : Demux  Outputs=3
  Demux6 : Demux  Outputs=2
  Gain : Gain  Gain=15/391
  Gain1 : Gain  Gain=15/11268
  Gain2 : Gain  Gain=15/(900000/391)
  Gain3 : Gain  Gain=15/(900000/11268)
  Gain4 : Gain  Gain=15/11268
  Gain5 : Gain  Gain=15/11268
  Gain6 : Gain  Gain=15/(900000/391)
  Gain7 : Gain  Gain=15/(900000/11268)
  Mux{,1,3..4} (4 alike) : Mux  Inputs=8
  Mux2 : Mux  Inputs=2
  Mux5 : Mux  Inputs=2
  Speed_System : Subsystem
  Speed_System1 : Subsystem
  Terminator{,1..3} (4 alike) : Terminator
  wires:
  Demux9/3 -> Mux3/8
  Demux9/2 -> Mux3/7
  Demux9/1 -> Mux3/6
  Gain6/1 -> Demux9/1
  Demux8/1 -> Mux3/5
  Gain7/1 -> Demux8/1
  Mains2_Current/1 -> Gain7/1
  Generator2_Current/1 -> Gain6/1
  Speed_System1/1(Out1) -> Mux1/6
  MPU2_speed/1 -> Speed_System1/1(In1)
  Generator2_Voltage/1 -> Gain4/1
  Mains2_Voltage/1 -> Gain5/1
  Gain4/1 -> Demux4/1
  Gain5/1 -> Demux5/1
  Demux7/1 -> Mux3/1
  Gain3/1 -> Demux7/1
  Mains1_Current/1 -> Gain3/1
  Demux3/3 -> Mux3/4
  Demux3/2 -> Mux3/3
  Demux3/1 -> Mux3/2
  Gain2/1 -> Demux3/1
  AnalogOut2/1 -> Terminator2/1
  AnalogOut3/1 -> Terminator3/1
  Demux6/1 -> AnalogOut2/1
  Demux6/2 -> AnalogOut3/1
  Mux3/1 -> Mux5/1
  Mux4/1 -> Mux5/2
  Mux5/1 -> Demux6/1
  Demux5/3 -> Mux1/4
  Demux5/2 -> Mux1/3
  Demux5/1 -> Mux1/2
  Demux4/3 -> Mux1/1
  Demux4/2 -> Mux/8
  Demux4/1 -> Mux/7
  Speed_System/1(Out1) -> Mux1/5
  Demux2/3 -> Mux/6
  Demux2/2 -> Mux/5
  Demux2/1 -> Mux/4
  Demux1/3 -> Mux/3
  Demux1/2 -> Mux/2
  Demux1/1 -> Mux/1
  AnalogOut/1 -> Terminator/1
  AnalogOut1/1 -> Terminator1/1
  Demux/1 -> AnalogOut/1
  Demux/2 -> AnalogOut1/1
  Generator1_Voltage/1 -> Gain/1
  Mux/1 -> Mux2/1
  Mux1/1 -> Mux2/2
  Mux2/1 -> Demux/1
  Mains1_Voltage/1 -> Gain1/1
  Gain/1 -> Demux1/1
  Gain1/1 -> Demux2/1
  Generator1_Current/1 -> Gain2/1
  MPU1_speed/1 -> Speed_System/1(In1)

== system generator_lib/Generator_09152015/Woodward Outputs ==
  Digital Output : Inport
  DIO Enable : Inport  Port=2
  Bias Enable : Inport  Port=3
  Bus Creator1 : BusCreator  Inputs=3
  DIO - Gr3 : Subsystem
  DIO - Woodward : Subsystem
  DOUT type config : Subsystem
  OpCtrl : rtio_opalrt_common/OpCtrl  CtrlName='OpCtrl'  boardid=0  BitstreamFilename=VC707_2-EX-0001-2_2_6_61-32AIO16DIO16DIOSel-01-01.bin  numconfig=-1  mode=Master  externalClock=off  decimRtsi=0  calibIO=off  SampleTime=0  loadinport=-1  BoardType=VC707  SecondaryPresent=off  sync_type=Audio
  PWM IO - Gr3 : Subsystem
  TSDIO - Gr3 : Subsystem
  Woodward Primary Inputs : Subsystem
  Error : Outport
  IDs : Outport  Port=2
  Digital Inputs : Outport  Port=3
  Gen1 Gov and AVR : Outport  Port=4
  Gen2 Gov and AVR : Outport  Port=5
  Gen1 Fuel Enable : Outport  Port=6
  Gen1 GCB : Outport  Port=7
  Gen1 MCB : Outport  Port=8
  Gen2 Fuel Enable : Outport  Port=9
  Gen2 GCB : Outport  Port=10
  Gen2 MCB : Outport  Port=11
  wires:
  DIO - Woodward/7(Gen2 MCB) -> Gen2 MCB/1
  DIO - Woodward/5(Gen2 Fuel Enable) -> Gen2 Fuel Enable/1
  DIO - Woodward/6(Gen2 GCB) -> Gen2 GCB/1
  DIO - Woodward/1(Gen1 Fuel Enable) -> Gen1 Fuel Enable/1
  DIO - Woodward/3(Gen1 MCB) -> Gen1 MCB/1
  DIO - Woodward/2(Gen1 GCB) -> Gen1 GCB/1
  Digital Output/1 -> TSDIO - Gr3/1(TSDout), PWM IO - Gr3/1(PWMOut), DIO - Woodward/2(Din_sim)
  Bias Enable/1 -> Woodward Primary Inputs/1(Bias-ctrl)
  Woodward Primary Inputs/2(Gen2 Gov and AVR) -> Gen2 Gov and AVR/1
  Woodward Primary Inputs/1(Gen1 Gov and AVR) -> Gen1 Gov and AVR/1
  DIO Enable/1 -> DIO - Woodward/4(control1), DIO - Woodward/3(control)
  Bus Creator1/1 -> Digital Inputs/1
  DIO - Gr3/1(DIn) -> DIO - Woodward/1(Din_Wood1), Bus Creator1/1  "DIN"
  TSDIO - Gr3/1(TSDin) -> Bus Creator1/2  "TSDIN"
  PWM IO - Gr3/1(PWMIn) -> Bus Creator1/3  "PWMIN"
  DIO - Woodward/4(DIn1) -> DIO - Gr3/1(Dout)
  OpCtrl/2 -> IDs/1
  OpCtrl/1 -> Error/1

== system generator_lib/1MVA Generator/GenSet_900kW_07232015/900kW Generator with  Primary Controllers ==
  wref : Inport
  Vtref : Inport  Port=2
  Enable : Inport  Port=3
  w_meas_Woodward : Inport  Port=4
  V_meas_Woodward : Inport  Port=5
  Woodward_Enable : Inport  Port=6
  Bus Creator1 : BusCreator
  Bus Creator3 : BusCreator  Inputs=3
  Bus Selector : BusSelector  OutputSignals=Vf_before,Vf_after
  Diesel Engine Speed & Voltage Control fast : Subsystem
  Synchronous Machine pu Fundamental : powerlib/Machines/Synchronous Machine pu Fundamental  PresetModel=22: 60Hz 460V 1075kVA 1800RPM  MechanicalLoad=Mechanical power Pm  ShowDetailedParameters=on  RotorType=Salient-pole  NominalParameters=[1.075e+006 460 60]  Stator=[0.01524 0.08 2.81 1.64]  Field=[0.004319 0.531]  Dampers2=[0.0652, 0.5134, 0.0287, 0.2553, 7.765e-3, 0.9167 ]  Dampers1=[0.2343 2.655 0.03365 0.2408]  Mechanical=[0.3222 0.01322 2]  PolePairs=2  InitialConditions="[ -99  0  0  0  0  0  0  0  0 ]"  SetSaturation=off  Saturation=[0.6404,0.7127,0.8441,0.9214,0.9956,1.082,1.19,1.316,1.457;0.7,0.7698,0.8872,0.9466,0.9969,1.046,1.1,1.151,1.201]  Units=per unit fundamental parameters  LoadFlowParameters=[1,0,0,0,0]  TsPowergui=0  TsBlock=-1  IterativeModel=Forward Euler  BusType=swing  Pref=0  Qref=0  Qmin=-inf  Qmax=inf  PLF=0  QLF=0
  A : PMIOPort  Port=1  Side=Right
  B : PMIOPort  Port=2  Side=Right
  C : PMIOPort  Port=3  Side=Right
  m : Outport
  Primary : Outport  Port=2
  wires:
  Woodward_Enable/1 -> Diesel Engine Speed & Voltage Control fast/7(Woodward Enable)
  Bus Creator3/1 -> Bus Creator1/2  "Vf"
  Bus Selector/2 -> Bus Creator3/3  "<Vf_after>"
  Bus Selector/1 -> Bus Creator3/2  "<Vf_before>"
  Diesel Engine Speed & Voltage Control fast/5(Misc) -> Bus Selector/1
  Bus Creator1/1 -> Primary/1
  Diesel Engine Speed & Voltage Control fast/4(w) -> Bus Creator1/4  "w"
  Diesel Engine Speed & Voltage Control fast/3(Vt) -> Bus Creator1/3  "vt"
  V_meas_Woodward/1 -> Diesel Engine Speed & Voltage Control fast/6(V_meas_Wood)
  w_meas_Woodward/1 -> Diesel Engine Speed & Voltage Control fast/5(w_meas_Wood)
  Synchronous Machine pu Fundamental/1 -> Diesel Engine Speed & Voltage Control fast/4(m), m/1
  Enable/1 -> Diesel Engine Speed & Voltage Control fast/3(Generator Enable)
  Diesel Engine Speed & Voltage Control fast/1(Pm) -> Bus Creator1/1, Synchronous Machine pu Fundamental/1  "Pm"
  Diesel Engine Speed & Voltage Control fast/2(Vf) -> Bus Creator3/1, Synchronous Machine pu Fundamental/2  "vf"
  wref/1 -> Diesel Engine Speed & Voltage Control fast/1(wref)
  Vtref/1 -> Diesel Engine Speed & Voltage Control fast/2(Vtref)
  connections:
  A/RConn1 -- Synchronous Machine pu Fundamental/RConn1
  B/RConn1 -- Synchronous Machine pu Fundamental/RConn2
  C/RConn1 -- Synchronous Machine pu Fundamental/RConn3

== system generator_lib/1MVA Generator/GenSet_900kW_07232015/Interface between Woodward Controller and simated generator ==
  note: Note: This may need a different scaling because it is the reference signal.
      | Reference has to be between 0.95 and 1.05 pu in order to be in tolerance.
  Woodward for wref : Inport
  Woodward for Vref : Inport  Port=2
  Add2 : Sum
  Add3 : Sum
  Gain2 : Gain
  Gain3 : Gain
  Mux1 : Mux  Inputs=2
  Vref_set : Constant  Value=0
  wref_set : Constant  Value=0
  wref,Vref : Outport
  wires:
  Woodward for Vref/1 -> Gain3/1
  Mux1/1 -> wref,Vref/1  "hardware"
  Woodward for wref/1 -> Gain2/1
  Add3/1 -> Mux1/2
  Vref_set/1 -> Add3/2
  Gain3/1 -> Add3/1  "bias"
  wref_set/1 -> Add2/2
  Add2/1 -> Mux1/1
  Gain2/1 -> Add2/1  "bias"

== system generator_lib/1MVA Generator/GenSet_900kW_07232015/NumOscillation ==
  Ground2 : powerlib/Elements/Ground  LConnTagsString=a
  "RLC " : powerlib/Elements/Parallel RLC Branch  LConnTagsString=a  RConnTagsString=__new0  BranchType=R  Resistance=10e6  Inductance=inf  SetiL0=off  InitialCurrent=0  Capacitance=10e-6  Setx0=off  InitialVoltage=0  Measurements=None
  RLC1 : powerlib/Elements/Parallel RLC Branch  LConnTagsString=a  RConnTagsString=__new0  BranchType=R  Resistance=10e6  Inductance=inf  SetiL0=off  InitialCurrent=0  Capacitance=10e-6  Setx0=off  InitialVoltage=0  Measurements=None
  RLC2 : powerlib/Elements/Parallel RLC Branch  LConnTagsString=a  RConnTagsString=__new0  BranchType=R  Resistance=10e6  Inductance=inf  SetiL0=off  InitialCurrent=0  Capacitance=10e-6  Setx0=off  InitialVoltage=0  Measurements=None
  RLC3 : powerlib/Elements/Parallel RLC Branch  LConnTagsString=a  RConnTagsString=__new0  BranchType=R  Resistance=10e-3  Inductance=inf  SetiL0=off  InitialCurrent=0  Capacitance=0  Setx0=off  InitialVoltage=0  Measurements=None
  RLC4 : powerlib/Elements/Parallel RLC Branch  LConnTagsString=a  RConnTagsString=__new0  BranchType=R  Resistance=10e-3  Inductance=inf  SetiL0=off  InitialCurrent=0  Capacitance=0  Setx0=off  InitialVoltage=0  Measurements=None
  RLC5 : powerlib/Elements/Parallel RLC Branch  LConnTagsString=a  RConnTagsString=__new0  BranchType=R  Resistance=10e-3  Inductance=inf  SetiL0=off  InitialCurrent=0  Capacitance=0  Setx0=off  InitialVoltage=0  Measurements=None
  A : PMIOPort  Port=1  Side=Left
  B : PMIOPort  Port=2  Side=Left
  C : PMIOPort  Port=3  Side=Left
  connections:
  "RLC "/RConn1 -- RLC1/RConn1 -- Ground2/LConn1 -- RLC2/RConn1
  "RLC "/LConn1 -- RLC5/RConn1
  RLC1/LConn1 -- RLC4/RConn1
  RLC3/RConn1 -- RLC2/LConn1
  A/RConn1 -- RLC3/LConn1
  B/RConn1 -- RLC4/LConn1
  C/RConn1 -- RLC5/LConn1

== system generator_lib/1MVA Generator/GenSet_900kW_07232015/Simulated Generator Controller 900 kW ==
  Pref : Inport
  Qref : Inport  Port=2
  mode : Inport  Port=3
  set_vtref : Inport  Port=4
  set_wref : Inport  Port=5
  gen_m : Inport  Port=6
  Bus Selector1 : BusSelector  OutputSignals="Output active power   Peo (pu),Output reactive power  Qeo (pu)"
  Multiport Switch : MultiPortSwitch  zeroidx=off
  Mux1 : Mux  Inputs=2
  Mux2 : Mux  Inputs=2
  Mux3 : Mux  Inputs=2
  PQ control : Subsystem
  PV control : Subsystem
  "wref, Vref" : Outport
  wires:
  Multiport Switch/1 -> "wref, Vref"/1
  mode/1 -> Multiport Switch/1
  Qref/1 -> PQ control/3(Q_ref (pu))
  set_wref/1 -> Mux3/1
  Bus Selector1/2 -> PQ control/4(Q (pu))  "<Output reactive power  Qeo (pu)>"
  Pref/1 -> PV control/1(P_ref (pu)), PQ control/1(P_ref (pu))
  Mux3/1 -> Multiport Switch/4
  Mux2/1 -> Multiport Switch/3
  Mux1/1 -> Multiport Switch/2
  set_vtref/1 -> Mux3/2, Mux2/2
  PV control/1(w_ref (pu)) -> Mux2/1
  PQ control/2(V_ref (pu)) -> Mux1/2
  PQ control/1(w_ref (pu)) -> Mux1/1
  gen_m/1 -> Bus Selector1/1
  Bus Selector1/1 -> PV control/2(P (pu)), PQ control/2(P (pu))  "<Output active power   Peo (pu)>"

== system generator_lib/1MVA Generator/GenSet_900kW_07232015/StabilityL ==
  Constant Load : powerlib/Elements/Three-Phase Parallel RLC Load  LConnTagsString=A|B|C  Configuration=Y (grounded)  NominalVoltage=v  NominalFrequency=60  ActivePower=kVA*1E3*pf  InductivePower=kVA*1E3*sqrt(1-pf^2)  CapacitivePower=0  Measurements=None  LoadType=constant Z
  A : PMIOPort  Port=1  Side=Left
  B : PMIOPort  Port=2  Side=Left
  C : PMIOPort  Port=3  Side=Left
  connections:
  C/RConn1 -- Constant Load/LConn3
  B/RConn1 -- Constant Load/LConn2
  A/RConn1 -- Constant Load/LConn1

== system generator_lib/1MVA Generator/Woodward Inputs/Speed_System ==
  In1 : Inport
  Clock1 : Clock
      settings: DisableCoverage=on
  Duty : Constant  DisableCoverage=on  Value=0.5
  Gain1 : Gain  Gain=5
  Gain3 : Gain  Gain=5
  Gain4 : Gain  Gain=1800
  Output : Trigonometry
  Product1 : Product  DisableCoverage=on  SaturateOnIntegerOverflow=on  InputSameDT=on  OutDataTypeStr=Inherit: Same as first input
  Product3 : Product  DisableCoverage=on  SaturateOnIntegerOverflow=on  InputSameDT=on  OutDataTypeStr=Inherit: Same as first input
  RTE Conversion : rteventslib/Signal Attributes/RTE Conversion  inputdatatype=RTE Boolean  outputdatatype=Double  compensation=Disabled  nbMaxEvents=10  sampleTime=Ts
  RTE SPWM : rteventslib/Sources/RTE SPWM  NumberPhases=1-ph  CenterAlignmentMode=On  MaxFreq=inf  MinFreq=0  EnablingPort=off  ComplementaryMode=off  SpaceVector=off  RiseTimeDelay=0  MaxEvents=10  SampleTime=Ts
  initialFreq : Constant  DisableCoverage=on  Value=2*pi
  Out1 : Outport
  wires:
  Product1/1 -> Output/1
  Clock1/1 -> Product1/1
  initialFreq/1 -> Product3/1
  Product3/1 -> Product1/2
  Gain4/1 -> Product3/2, RTE SPWM/1
  Output/1 -> Gain3/1
  In1/1 -> Gain4/1
  RTE SPWM/1 -> RTE Conversion/1
  Duty/1 -> RTE SPWM/2
  RTE Conversion/1 -> Gain1/1
  Gain1/1 -> Out1/1

== system generator_lib/1MVA Generator/Woodward Outputs/DIO - Gr3 ==
  Dout : Inport
  Bus Creator : BusCreator  Inputs=2
  Bus Selector : BusSelector  OutputSignals=DI_CH00-07  OutputAsBus=on
  Bus Selector1 : BusSelector  OutputSignals=DI_CH08-15  OutputAsBus=on
  Conditioning : Subsystem
  Conditioning1 : Subsystem
  DigitalIn : rtio_opalrt_common/DigitalIn  CtrlName='OpCtrl'  portNb=5  FcnNos=Slot 3 Module A Subsection 1  size=1  maxcount=-2  count=8  sampleTime=0  numchan=8
      settings: AttributesFormatString=%<CtrlName>
  DigitalIn1 : rtio_opalrt_common/DigitalIn  CtrlName='OpCtrl'  portNb=6  FcnNos=Slot 3 Module A Subsection 2  size=1  maxcount=-2  count=8  sampleTime=0  numchan=8
      settings: AttributesFormatString=%<CtrlName>
  DigitalOut : rtio_opalrt_common/DigitalOut  CtrlName='OpCtrl'  portNb=5  FcnNos=Slot 3 Module B Subsection 1  size=1  maxcount=-2  count=8  numchan=8
      settings: AttributesFormatString=%<CtrlName>
  DigitalOut1 : rtio_opalrt_common/DigitalOut  CtrlName='OpCtrl'  portNb=6  FcnNos=Slot 3 Module B Subsection 2  size=1  maxcount=-2  count=8  numchan=8
      settings: AttributesFormatString=%<CtrlName>
  Terminator{1,3,5..6} (4 alike) : Terminator
  DIn : Outport
  wires:
  Conditioning1/1(Out1) -> Bus Creator/2
  Conditioning/1(Out1) -> Bus Creator/1
  Bus Creator/1 -> DIn/1
  DigitalIn1/1 -> Conditioning1/1(In1)  "DI_CH08-15"
  DigitalIn/1 -> Conditioning/1(In1)  "DI_CH00-07"
  DigitalIn1/2 -> Terminator6/1
  DigitalIn/2 -> Terminator5/1
  Bus Selector1/1 -> DigitalOut1/1
  Bus Selector/1 -> DigitalOut/1
  Dout/1 -> Bus Selector1/1, Bus Selector/1
  DigitalOut1/1 -> Terminator1/1
  DigitalOut/1 -> Terminator3/1

== system generator_lib/1MVA Generator/Woodward Outputs/DIO - Woodward ==
  note: These are the inputs to
      | the HIL Outputs.
  Din_wood : Inport
  Din_sim : Inport  Port=2
  control : Inport  Port=3
  Add : Sum
  Add1 : Sum
  Bus Creator : BusCreator  Inputs=2
  Bus Selector1 : BusSelector  OutputSignals=16 DOUT GR3.08-11.signal1,16 DOUT GR3.08-11.signal2,16 DOUT GR3.08-11.signal3,16 DOUT GR3.08-11.signal4,16 DOUT GR3.12-15.signal1,16 DOUT GR3.12-15.signal2,16 DOUT GR3.12-15.signal3,16 DOUT GR3.12-15.signal4
  Bus Selector2 : BusSelector  OutputSignals=16 DOUT GR3.00-03.Estop,16 DOUT GR3.00-03.Start_Auto,16 DOUT GR3.00-03.ExtAlarm,16 DOUT GR3.00-03.EnableMCB,16 DOUT GR3.04-07.MCBOpen,16 DOUT GR3.04-07.GCBOpen,16 DOUT GR3.04-07.signal3,16 DOUT GR3.04-07.signal4
  Bus Selector3 : BusSelector  OutputSignals=DI_CH00-07.Close_GCB,DI_CH00-07.Open_GCB,DI_CH00-07.Close_MCB,DI_CH08-15.Open_MCB
  Bus Selector4 : BusSelector  OutputSignals=16 DOUT GR3.04-07.MCBOpen,16 DOUT GR3.04-07.GCBOpen
  Compare To Zero{,1..4} (5 alike) : simulink/Logic and Bit Operations/Compare To Zero  relop=>  OutDataTypeStr=boolean
  Constant : Constant
  Mux : Mux  Inputs=8
  Mux1 : Mux  Inputs=8
  S-R Flip-Flop : simulink_extras/Flip Flops/S-R Flip-Flop  initial_condition=1
  S-R Flip-Flop1 : simulink_extras/Flip Flops/S-R Flip-Flop  initial_condition=1
  Switch{1..4} (4 alike) : Switch  Threshold=0.5
  GCB : Outport
  MCB : Outport  Port=2
  DIn : Outport  Port=3
  wires:
  Constant/1 -> Add1/1, Add/2
  Add1/1 -> MCB/1
  Add/1 -> GCB/1
  Bus Selector2/2 -> Mux/2  "<Start_Auto>"
  Bus Selector2/3 -> Mux/3  "<ExtAlarm>"
  S-R Flip-Flop1/2 -> Switch4/1
  S-R Flip-Flop/2 -> Switch3/1
  Bus Selector1/2 -> Switch4/3  "<signal2>"
  Bus Selector1/1 -> Switch3/3  "<signal1>"
  Bus Selector2/7 -> Mux/7  "<signal3>"
  Switch3/1 -> Mux1/2
  Switch4/1 -> Mux1/1
  Mux1/1 -> Bus Creator/2  "DI_CH08-15"
  Bus Selector1/8 -> Mux1/8  "<signal4>"
  Bus Selector1/7 -> Mux1/7  "<signal3>"
  Bus Selector1/6 -> Mux1/6  "<signal2>"
  Bus Selector1/5 -> Mux1/5  "<signal1>"
  Bus Selector1/4 -> Mux1/4  "<signal4>"
  Bus Selector1/3 -> Mux1/3  "<signal3>"
  Bus Selector2/8 -> Mux/8  "<signal4>"
  Switch2/1 -> Add1/2, Mux/5
  Compare To Zero2/1 -> Switch4/2, Switch3/2, Switch2/2, Switch1/2
  Bus Selector3/1 -> Compare To Zero1/1  "<Close_GCB>"
  S-R Flip-Flop1/1 -> Switch2/1
  Compare To Zero3/1 -> S-R Flip-Flop1/1
  Bus Selector3/4 -> Compare To Zero3/1  "<Open_MCB>"
  Compare To Zero4/1 -> S-R Flip-Flop1/2
  Bus Selector3/3 -> Compare To Zero4/1  "<Close_MCB>"
  Bus Selector4/2 -> Switch1/3  "<GCBOpen>"
  Compare To Zero1/1 -> S-R Flip-Flop/2
  Compare To Zero/1 -> S-R Flip-Flop/1
  Bus Selector3/2 -> Compare To Zero/1  "<Open_GCB>"
  Switch1/1 -> Add/1, Mux/6
  S-R Flip-Flop/1 -> Switch1/1
  Bus Creator/1 -> DIn/1
  control/1 -> Compare To Zero2/1
  Mux/1 -> Bus Creator/1  "DI_CH00-07"
  Bus Selector2/4 -> Mux/4  "<EnableMCB>"
  Bus Selector2/1 -> Mux/1  "<Estop>"
  Bus Selector4/1 -> Switch2/3  "<MCBOpen>"
  Din_sim/1 -> Bus Selector1/1, Bus Selector2/1, Bus Selector4/1
  Din_wood/1 -> Bus Selector3/1

== system generator_lib/1MVA Generator/Woodward Outputs/DOUT type config ==
  note: The Constants are used to select Digital Output type:
      | - 0: Time-Stamped Digital Output
      | - 1: Pulse-Width Modulated DIgital Output
  DataIn Send : rtio_opalrt_common/DataIn Send  CtrlName='OpCtrl'  FcnNos=11  width=1  portType=double  checkVersion=off  expectedId=0  expectedVersion=0  opComp=>=
      settings: AttributesFormatString=%<CtrlName>
  DataIn Send1 : rtio_opalrt_common/DataIn Send  CtrlName='OpCtrl'  FcnNos=12  width=1  portType=double  checkVersion=off  expectedId=0  expectedVersion=0  opComp=>=
      settings: AttributesFormatString=%<CtrlName>
  Subsection 3 DOUT type : Constant
  Subsection 4 DOUT type : Constant
  Terminator1 : Terminator
  Terminator2 : Terminator
  wires:
  DataIn Send/1 -> Terminator2/1
  DataIn Send1/1 -> Terminator1/1
  Subsection 4 DOUT type/1 -> DataIn Send1/1
  Subsection 3 DOUT type/1 -> DataIn Send/1

== system generator_lib/1MVA Generator/Woodward Outputs/PWM IO - Gr3 ==
  PWMOut : Inport
  Bus Creator : BusCreator  Inputs=2
  Bus Creator1 : BusCreator  Inputs=2
  Bus Creator2 : BusCreator  Inputs=2
  Bus Selector : BusSelector  OutputSignals=FreqPWMOut16-23,DutyPWMOut16-23
  Bus Selector1 : BusSelector  OutputSignals=FreqPWMOut24-31,DutyPWMOut24-31
  Bus Selector2 : BusSelector  OutputSignals=16 PWMOUT GR3.Ch16-23,16 PWMOUT GR3.Ch24-31
  PWM In : rtio_opalrt_common/PWM In  CtrlName='OpCtrl'  portNb=9  FcnNos=Slot 3 Module A Subsection 3  maxCount=8  Count=8  sampleTime=0  numchan=8
      settings: AttributesFormatString=%<CtrlName>
  PWM In1 : rtio_opalrt_common/PWM In  CtrlName='OpCtrl'  portNb=10  FcnNos=Slot 3 Module A Subsection 4  maxCount=8  Count=8  sampleTime=0  numchan=8
      settings: AttributesFormatString=%<CtrlName>
  PWM Out : rtio_opalrt_common/PWM Out  CtrlName='OpCtrl'  portNb=9  FcnNos=Slot 3 Module B Subsection 3  size=64  maxcount=8  count=8  polarity=Active High  symMode=Symmetric  complementary=off  deadTime=0  numchan=8  loadnb=1  initphase=[0 0 0 0 0 0 0 0]
      settings: AttributesFormatString=%<CtrlName>
  PWM Out1 : rtio_opalrt_common/PWM Out  CtrlName='OpCtrl'  portNb=10  FcnNos=Slot 3 Module B Subsection 4  size=64  maxcount=8  count=8  polarity=Active High  symMode=Symmetric  complementary=off  deadTime=0  numchan=8  loadnb=2  initphase=[0 0 0 0 0 0 0 0]
      settings: AttributesFormatString=%<CtrlName>
  Terminator{,1,4..5} (4 alike) : Terminator
  PWMIn : Outport
  wires:
  Bus Selector2/2 -> Bus Selector1/1  "<Ch24-31>"
  PWM In1/2 -> Bus Creator2/2  "Duty"
  PWM In1/1 -> Bus Creator2/1  "Freq"
  PWM In/2 -> Bus Creator1/2  "Duty"
  PWM In/1 -> Bus Creator1/1  "Freq"
  PWM In/3 -> Terminator4/1
  PWM In1/3 -> Terminator5/1
  Bus Creator2/1 -> Bus Creator/2  "PWMI_CH24-31"
  Bus Creator1/1 -> Bus Creator/1  "PWMI_CH16-23"
  Bus Creator/1 -> PWMIn/1
  Bus Selector2/1 -> Bus Selector/1  "<Ch16-23>"
  PWMOut/1 -> Bus Selector2/1
  PWM Out1/1 -> Terminator1/1
  Bus Selector1/2 -> PWM Out1/2  "<DutyPWMOut24-31>"
  Bus Selector1/1 -> PWM Out1/1  "<FreqPWMOut24-31>"
  PWM Out/1 -> Terminator/1
  Bus Selector/2 -> PWM Out/2  "<DutyPWMOut16-23>"
  Bus Selector/1 -> PWM Out/1  "<FreqPWMOut16-23>"
